simulink model "pacemaker_ass2_test"  (R2017b)
settings: Solver=FixedStepAuto  StartTime=0.0  StopTime=inf  FixedStep=0.001  RelTol=1e-3  EnableMultiTasking=on
libraries: frdmk64flib x3
settings Model: ExtModeTrigDuration=5  Creator=montema2  LastModifiedBy=huy62
settings SolverCC: AutoInsertRateTranBlk=on
settings DataIOCC: LimitDataPoints=on
settings OptimizationCC: PassReuseOutputArgsAs=Individual arguments  MaxStackSize=64
settings DebuggingCC: ParameterTunabilityLossMsg=error  AllowSymbolicDim=off  SFUnexpectedBacktrackingDiag=warning  SFNoUnconditionalDefaultTransitionDiag=warning  SFExecutionAtInitializationDiag=none
settings HardwareCC: ProdBitPerPointer=32  ProdBitPerSizeT=32  ProdBitPerPtrDiffT=32  ProdLargestAtomicInteger=Long  ProdLargestAtomicFloat=Double  ProdWordSize=32  ProdHWDeviceType=ARM Compatible->ARM Cortex
settings SFSimCC: MATLABDynamicMemAlloc=off
settings RTWCC: SystemTargetFile=ert.tlc  HardwareBoard=NXP FRDM-K64F  TemplateMakefile=ert_default_tmf  GenerateReport=on  Toolchain=GNU Tools for ARM Embedded Processors  IncludeHyperlinkInReport=on  LaunchReport=on  GenerateTraceInfo=on  GenerateTraceReport=on  GenerateTraceReportSl=on  GenerateTraceReportSf=on  GenerateTraceReportEml=on
settings CodeAppCC: ForceParamTrailComments=on  IgnoreCustomStorageClasses=off  OperatorAnnotations=on  SimulinkDataObjDesc=on  SFDataObjDesc=on  InsertBlockDesc=on
settings ConfigComp: CovMetricSettings=dw  CovHtmlReporting=on  CovSaveCumulativeToWorkspaceVar=on  CovSaveSingleToWorkspaceVar=on  CovShowResultsExplorer=off  CovExternalEMLEnable=off  CovSFcnEnable=off

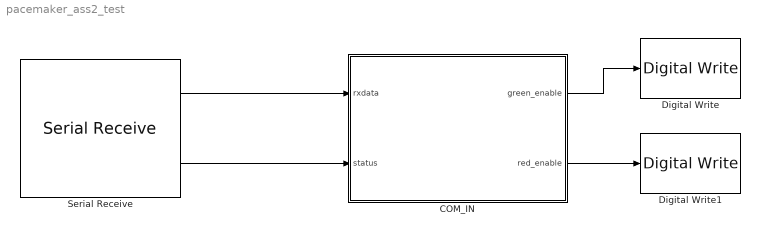
== system pacemaker_ass2_test ==
  COM_IN : Stateflow chart  TreatAsAtomicUnit=on
  Digital Write : frdmk64flib/Digital Write  Whichpin=GREEN_LED
      settings: SourceProductName=Simulink Coder Support Package for NXP FRDM-K64F Board
  Digital Write1 : frdmk64flib/Digital Write  Whichpin=RED_LED
      settings: SourceProductName=Simulink Coder Support Package for NXP FRDM-K64F Board
  Serial Receive : frdmk64flib/Serial Receive  SCIModule=0  Baudrate=uint32(9600)  Parity=None  StopBits=1  HardwareFlowControl=None  ByteOrder=LittleEndian  DataType=uint8  DataLength=2  BlockingMode=off  OutputStatus=on  SampleTime=-1
      settings: SourceProductName=Simulink Coder Support Package for NXP FRDM-K64F Board
  wires:
  Serial Receive/2 -> COM_IN/2(status)
  COM_IN/1(green_enable) -> Digital Write/1
  Serial Receive/1 -> COM_IN/1(rxdata)
  COM_IN/2(red_enable) -> Digital Write1/1

== stateflow chart pacemaker_ass2_test/COM_IN ==
  settings: executeAtInitialization=1
  state INITIAL
    entry:
    red_enable = 0;
    green_enable = 0;
  state STANDBY
    entry:
    green_enable = 0;
    red_enable = 0;
  state state
    entry:
    green_enable = 0;
    red_enable = 1;
  state state2
    entry:
    red_enable = 0;
    green_enable = 1;
  state -> STANDBY : [after(500,msec)]
  (default) -> INITIAL
  INITIAL -> STANDBY
  STANDBY -> (junction 11) : [status == 0]
  (junction 11) -> state [order 1] : [rxdata(1) == 22 && rxdata(2) == 4]
  (junction 11) -> STANDBY [order 3]
  (junction 11) -> state2 [order 2] : [rxdata(2) == 14]
  state2 -> STANDBY : [after(500,msec)]
  data: rxdata input uint8; status input uint8; green_enable output; yes local; red_enable output
